simulink model "Q5"  (R2018b)
settings: Solver=VariableStepAuto  StartTime=0.0  StopTime=20  RelTol=1e-3
values from neighbouring files (symbols this model uses):
  A = [0      0      0      1      0      0 ... (first row only)    [load_parameter.m]    (also in parameter.m)
  B = [0      0 ... (first row only)    [load_parameter.m]    (also in parameter.m)
  C = [1   0   0   0   0   0 ... (first row only)    [load_parameter.m]    (also in parameter.m)
  K51 = K5(:,1:6)    [main.m]
  K52 = K5(:,7:9)    [main.m]
  x0 = [0.2;  -0.1;   0.15;  -1;  0.8;   0]    [load_parameter.m]    (also in parameter.m)
  ysp = -0.1*C/A*B*[-0.5+(3-1)/20; 0.1+(1-1)/(3+5+10)]    [main.m]
undefined symbols (not defined in the file or in its folder): L5
settings Model: Creator=nmzxc  LastModifiedBy=nmzxc

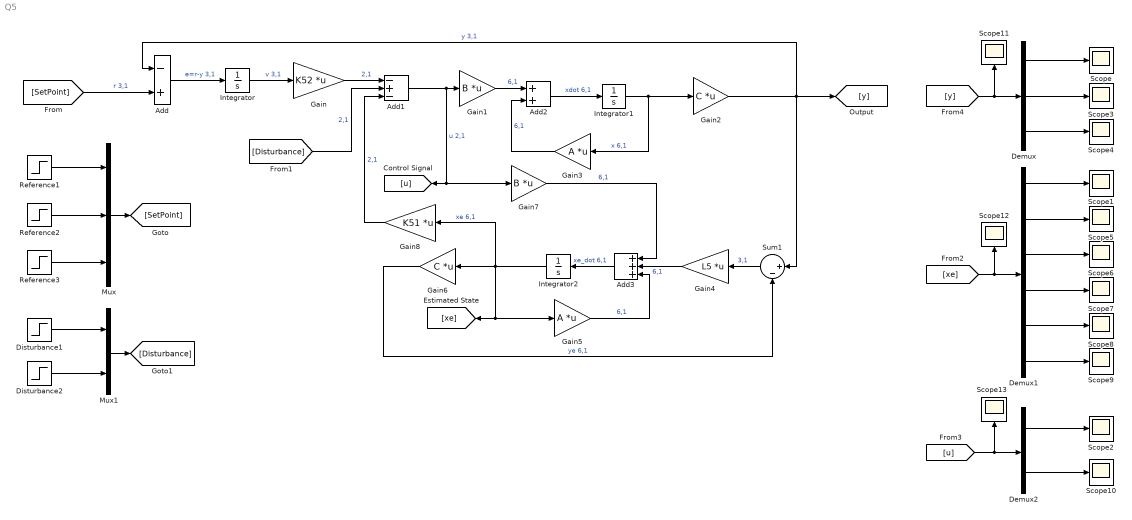
== system Q5 ==
  Add : Sum  Inputs=-+
  Add1 : Sum  Inputs=-+-
  Add2 : Sum
  Add3 : Sum  Inputs=+++
  Demux : Demux  Outputs=3
  Demux1 : Demux  Outputs=6
  Demux2 : Demux  Outputs=2
  Disturbance1 : Step  Time=10  After=-1  SampleTime=0
  Disturbance2 : Step  Time=10  SampleTime=0
  Gain : Gain  Gain=K52  Multiplication=Matrix(K*u) (u vector)
  Gain1 : Gain  Gain=B  Multiplication=Matrix(K*u) (u vector)
  Gain2 : Gain  Gain=C  Multiplication=Matrix(K*u) (u vector)
  Gain3 : Gain  Gain=A  Multiplication=Matrix(K*u) (u vector)
  Gain4 : Gain  Gain=L5  Multiplication=Matrix(K*u) (u vector)
  Gain5 : Gain  Gain=A  Multiplication=Matrix(K*u) (u vector)
  Gain6 : Gain  Gain=C  Multiplication=Matrix(K*u) (u vector)
  Gain7 : Gain  Gain=B  Multiplication=Matrix(K*u) (u vector)
  Gain8 : Gain  Gain=K51  Multiplication=Matrix(K*u) (u vector)
  Integrator : Integrator
  Integrator1 : Integrator  InitialCondition=x0
  Integrator2 : Integrator
  Mux : Mux  Inputs=3
  Mux1 : Mux  Inputs=2
  Reference1 : Step  Time=0  After=ysp(1)  SampleTime=0
  Reference2 : Step  Time=0  After=ysp(2)  SampleTime=0
  Reference3 : Step  Time=0  After=ysp(3)  SampleTime=0
  Scope{,1..13} (14 alike) : Scope
  Sum1 : Sum  Inputs=|+-
  wires:
  Add1/1 -> [u], Gain7/1, Gain1/1  "u 2,1"
  Gain1/1 -> Add2/1  "6,1"
  Add2/1 -> Integrator1/1  "xdot 6,1"
  Integrator1/1 -> Gain3/1, Gain2/1  "x 6,1"
  Gain3/1 -> Add2/2  "6,1"
  Gain2/1 -> Sum1/1, [y], Add/1  "y 3,1"
  Sum1/1 -> Gain4/1  "3,1"
  Add3/1 -> Integrator2/1  "xe_dot 6,1"
  Integrator2/1 -> Gain8/1, Gain6/1, [xe], Gain5/1  "xe 6,1"
  Gain6/1 -> Sum1/2  "ye 6,1"
  Gain5/1 -> Add3/3  "6,1"
  Gain4/1 -> Add3/2  "6,1"
  Gain7/1 -> Add3/1  "6,1"
  Integrator/1 -> Gain/1  "v 3,1"
  Add/1 -> Integrator/1  "e=r-y 3,1"
  Gain/1 -> Add1/1  "2,1"
  [SetPoint] -> Add/2  "r 3,1"
  Reference1/1 -> Mux/1
  Reference2/1 -> Mux/2
  Reference3/1 -> Mux/3
  Mux/1 -> [SetPoint]
  Disturbance1/1 -> Mux1/1
  Disturbance2/1 -> Mux1/2
  Mux1/1 -> [Disturbance]
  Gain8/1 -> Add1/3  "2,1"
  [Disturbance] -> Add1/2  "2,1"
  [u] -> Scope13/1, Demux2/1
  [y] -> Scope11/1, Demux/1
  Demux/1 -> Scope/1
  Demux/2 -> Scope3/1
  Demux/3 -> Scope4/1
  Demux1/2 -> Scope5/1
  Demux1/3 -> Scope6/1
  Demux1/1 -> Scope1/1
  Demux1/4 -> Scope7/1
  Demux1/5 -> Scope8/1
  Demux1/6 -> Scope9/1
  Demux2/1 -> Scope2/1
  Demux2/2 -> Scope10/1
  [xe] -> Scope12/1, Demux1/1
